simulink model "p3_mdl"  (R2021b)
settings: Solver=VariableStepAuto  StartTime=0.0  StopTime=10.0  RelTol=1e-6
values from neighbouring files (symbols this model uses):
  alpha = 0.2    [p3.m]
settings Model: Creator=Tomo  LastModifiedBy=Tomo

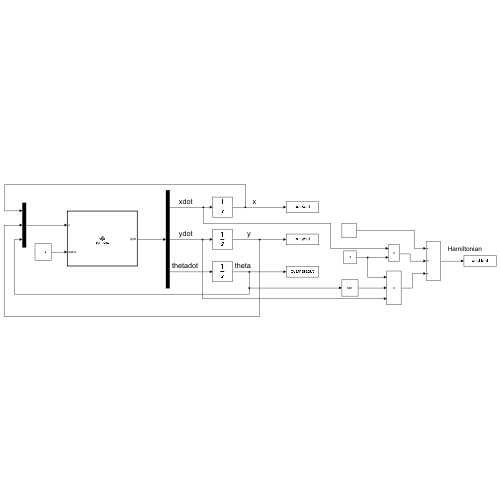
[thumbnail: Simulink's stored preview of the top-level diagram]
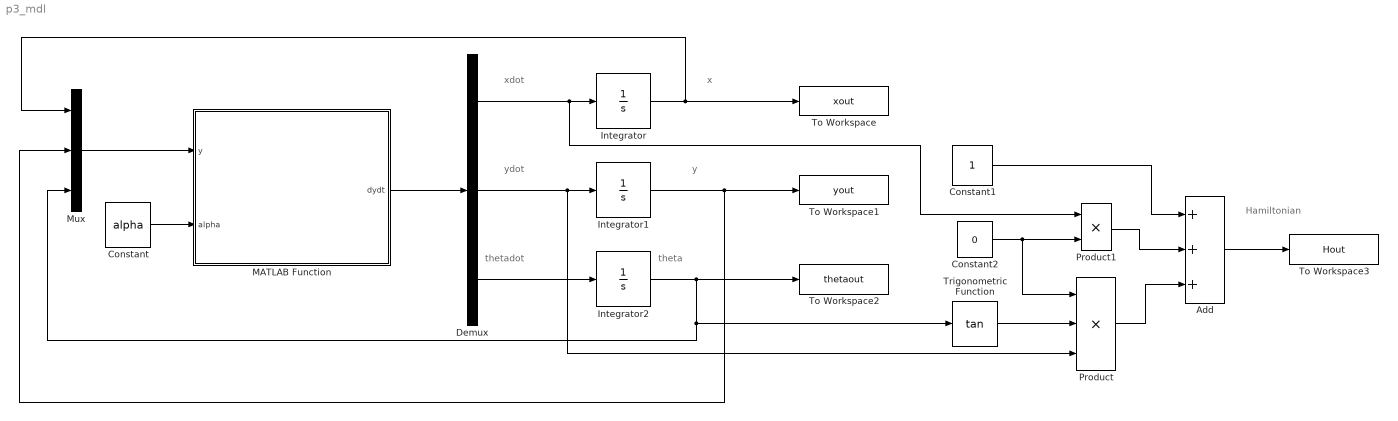
== system p3_mdl ==
  note: Hamiltonian
  note: xdot
  note: ydot
  note: thetadot
  note: x
  note: y
  note: theta
  Add : Sum  Inputs=+++
  Constant : Constant  Value=alpha
  Constant1 : Constant
  Constant2 : Constant  Value=0
  Demux : Demux  Outputs=3
  Integrator : Integrator  InitialCondition=1
  Integrator1 : Integrator  InitialCondition=1
  Integrator2 : Integrator  InitialCondition=1.5708
  MATLAB Function : MATLAB Function  TreatAsAtomicUnit=on
  Mux : Mux  Inputs=3
  Product : Product  Inputs=3
  Product1 : Product
  To Workspace : ToWorkspace  VariableName=xout  SaveFormat=Structure  SampleTime=-1
      settings: Save2DSignal=2-D array (concatenate along first dimension)
  To Workspace1 : ToWorkspace  VariableName=yout  SaveFormat=Structure  SampleTime=-1
      settings: Save2DSignal=2-D array (concatenate along first dimension)
  To Workspace2 : ToWorkspace  VariableName=thetaout  SaveFormat=Structure  SampleTime=-1
      settings: Save2DSignal=2-D array (concatenate along first dimension)
  To Workspace3 : ToWorkspace  VariableName=Hout  SaveFormat=Structure  SampleTime=-1
      settings: Save2DSignal=2-D array (concatenate along first dimension)
  Trigonometric Function : Trigonometry  Operator=tan
  wires:
  MATLAB Function/1(dydt) -> Demux/1
  Demux/3 -> Integrator2/1
  Demux/2 -> Product/3, Integrator1/1
  Demux/1 -> Product1/1, Integrator/1
  Mux/1 -> MATLAB Function/1(y)
  Constant/1 -> MATLAB Function/2(alpha)
  Constant2/1 -> Product1/2, Product/1
  Trigonometric Function/1 -> Product/2
  Constant1/1 -> Add/1
  Product1/1 -> Add/2
  Product/1 -> Add/3
  Add/1 -> To Workspace3/1
  Integrator/1 -> To Workspace/1, Mux/1
  Integrator1/1 -> To Workspace1/1, Mux/2
  Integrator2/1 -> To Workspace2/1, Mux/3, Trigonometric Function/1

== matlab function p3_mdl/MATLAB Function ==
  data: y input; dydt output; alpha input
function dydt = sys_ode(y, alpha)
%{
    Function: sys_ode
    ------------------
    ODE representation of the optimal control problem of problem 3 hw5.

    args: 
        t: time 
        y: state variables        
        alpha: constant (known parameter)
    returns:
        derivative of the state variables 
%}
    dydt = zeros(3,1);
    u = -alpha * (3 * y(2) - y(2)^3);
    dydt(1) = cos(y(3)) + u;
    dydt(2) = sin(y(3));
    dydt(3) = 3 * alpha * (1 - y(2)^2) * cos(y(3))^2;
end
